simulink model "Main_Sim_test_rwafail_mtqfail"  (R2018b)
settings: Solver=FixedStepAuto  StartTime=0.0  StopTime=30000  FixedStep=simParams.sample_time_s  RelTol=1e-3  EnableMultiTasking=on
undefined symbols (not defined in the file): FSW_Lib
libraries: actuators_lib x1, CDH_command_lib x1, Environment_lib x1, MEKF_SensorCheck_Lib x1, actuator_processing_lib x1, allocation_lib x1, control_command_generation_lib x1, evironmentEstimation_lib x1, mode_select_lib x1, target_gen_lib x1, Sensors_Lib x1, satelliteDynamics_lib x1
settings Model: Creator=devantormey  LastModifiedBy=colem
settings OptimizationCC: LifeSpan=inf
settings DebuggingCC: SFUnexpectedBacktrackingDiag=warning  SFNoUnconditionalDefaultTransitionDiag=warning
settings SFSimCC: SimUseLocalCustomCode=off
settings RTWCC: RTWUseLocalCustomCode=off
settings CodeAppCC: StateflowObjectComments=on
settings GRTTargetCC: TargetLangStandard=C89/C90 (ANSI)  GeneratePreprocessorConditionals=Disable all
settings ConfigComp: CovMetricSettings=dw  CovHtmlReporting=on  CovSaveCumulativeToWorkspaceVar=on  CovSaveSingleToWorkspaceVar=on  CovExternalEMLEnable=off

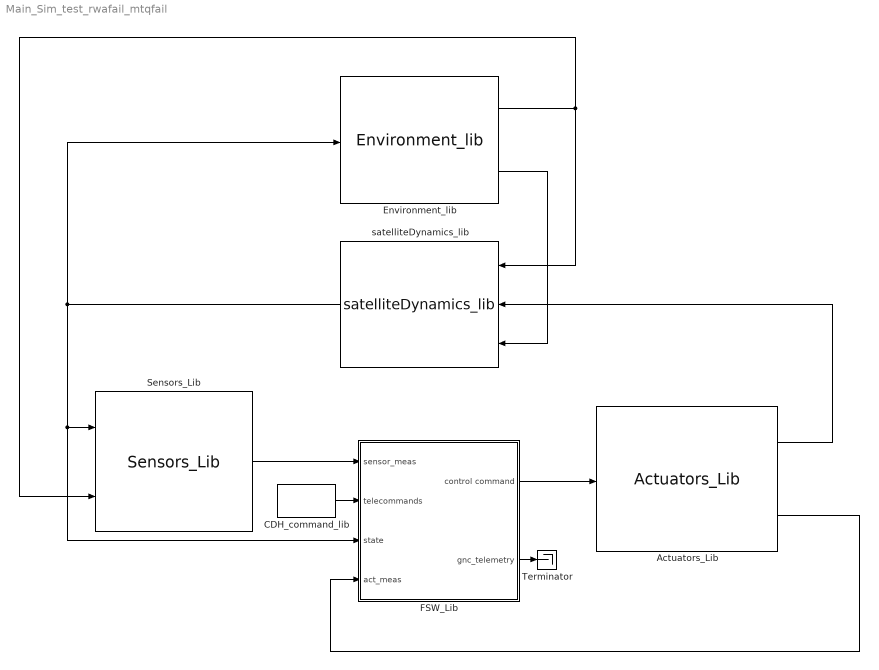
== system Main_Sim_test_rwafail_mtqfail ==
  Actuators_Lib : actuators_lib/Actuators_Lib  SystemSampleTime=-1
  CDH_command_lib : CDH_command_lib/CDH_command_lib  SystemSampleTime=-1
  Environment_lib : Environment_lib/Environment_lib  SystemSampleTime=-1
  FSW_Lib : Subsystem  AncestorBlock=FSW_Lib/FSW_Lib
  Sensors_Lib : Sensors_Lib/Sensors_Lib  SystemSampleTime=-1
      link override Goto3: GotoTag=B_eci_T
  Terminator : Terminator
  satelliteDynamics_lib : satelliteDynamics_lib/satelliteDynamics_lib  SystemSampleTime=-1
      link override "RigidBodyDynamics/Discrete-Time Integrator ": InitialCondition=simParams.initialConditions.w0
  wires:
  FSW_Lib/1(control command) -> Actuators_Lib/1
  Sensors_Lib/1 -> FSW_Lib/1(sensor_meas)
  satelliteDynamics_lib/1 -> Environment_lib/1, FSW_Lib/3(state), Sensors_Lib/1
  Environment_lib/1 -> Sensors_Lib/2, satelliteDynamics_lib/1
  Actuators_Lib/1 -> satelliteDynamics_lib/2
  FSW_Lib/2(gnc_telemetry) -> Terminator/1
  CDH_command_lib/1 -> FSW_Lib/2(telecommands)
  Environment_lib/2 -> satelliteDynamics_lib/3
  Actuators_Lib/2 -> FSW_Lib/4(act_meas)

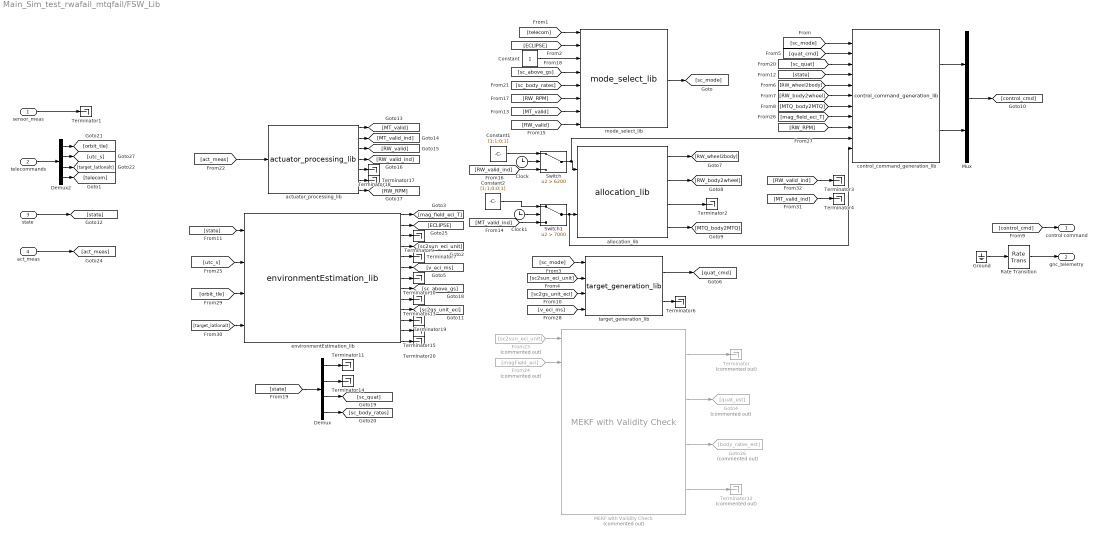
== system Main_Sim_test_rwafail_mtqfail/FSW_Lib ==
  sensor_meas : Inport
  telecommands : Inport  Port=2
  state : Inport  Port=3
  act_meas : Inport  Port=4
  Clock : Clock
  Clock1 : Clock
  Constant : Constant
  Constant1 : Constant  Value=[1;1;0;1]
  Constant2 : Constant  Value=[1;1;0;0;1]
  Demux : Demux  Outputs=[3 3 4 3]
  Demux2 : Demux  Outputs=[9 1 3 7]
  From23 : From  Commented=on  GotoTag=sc2sun_eci_unit
  From24 : From  Commented=on  GotoTag=magField_eci
  Goto26 : Goto  Commented=on  GotoTag=body_rates_est
  Goto4 : Goto  Commented=on  GotoTag=quat_est
  Ground : Ground
  MEKF with Validity Check : MEKF_SensorCheck_Lib/MEKF with Validity Check  Commented=on  SystemSampleTime=-1
  Mux : Mux  Inputs=[4 5]
  Rate Transition : RateTransition  OutPortSampleTime=fswParams.sample_time_s
  Switch : Switch  Criteria=u2 > Threshold  Threshold=6200
  Switch1 : Switch  Criteria=u2 > Threshold  Threshold=7000
  Terminator : Terminator  Commented=on
  Terminator{1..4,6..7,9..11,13..15,17..20} (16 alike) : Terminator
  Terminator12 : Terminator  Commented=on
  actuator_processing_lib : actuator_processing_lib/actuator_processing_lib  SystemSampleTime=-1
  allocation_lib : allocation_lib/allocation_lib  SystemSampleTime=-1
  control_command_generation_lib : control_command_generation_lib/control_command_generation_lib  SystemSampleTime=-1
  environmentEstimation_lib : evironmentEstimation_lib/environmentEstimation_lib  SystemSampleTime=-1
  mode_select_lib : mode_select_lib/mode_select_lib  SystemSampleTime=-1
  target_generation_lib : target_gen_lib/target_generation_lib  SystemSampleTime=-1
  control command : Outport
  gnc_telemetry : Outport  Port=2
  wires:
  [MT_valid_ind] -> Terminator4/1
  [RW_valid_ind] -> Terminator3/1
  Rate Transition/1 -> gnc_telemetry/1
  target_generation_lib/1 -> [quat_cmd]
  [target_latlonalt] -> environmentEstimation_lib/4
  Demux2/3 -> [target_latlonalt]
  Demux2/1 -> [orbit_tle]
  [v_eci_ms] -> target_generation_lib/4
  [RW_RPM] -> control_command_generation_lib/9
  [mag_field_eci_T] -> control_command_generation_lib/8
  Demux2/2 -> [utc_s]
  Demux2/4 -> [telecom]
  MEKF with Validity Check/2 -> Goto4/1
  MEKF with Validity Check/3 -> Goto26/1
  MEKF with Validity Check/4 -> Terminator12/1
  MEKF with Validity Check/1 -> Terminator/1
  From24/1 -> MEKF with Validity Check/2
  From23/1 -> MEKF with Validity Check/1
  environmentEstimation_lib/11 -> Terminator19/1
  environmentEstimation_lib/13 -> Terminator20/1
  environmentEstimation_lib/12 -> Terminator15/1
  Demux/2 -> Terminator14/1
  Demux/1 -> Terminator11/1
  Demux/4 -> [sc_body_rates]
  Demux/3 -> [sc_quat]
  [state] -> Demux/1
  [act_meas] -> actuator_processing_lib/1
  actuator_processing_lib/7 -> [RW_RPM]
  actuator_processing_lib/6 -> Terminator17/1
  actuator_processing_lib/5 -> Terminator18/1
  actuator_processing_lib/4 -> [RW_valid_ind]
  actuator_processing_lib/3 -> [RW_valid]
  actuator_processing_lib/2 -> [MT_valid_ind]
  actuator_processing_lib/1 -> [MT_valid]
  act_meas/1 -> [act_meas]
  [state] -> control_command_generation_lib/4
  [state] -> environmentEstimation_lib/1
  state/1 -> [state]
  [sc2gs_unit_eci] -> target_generation_lib/3
  [orbit_tle] -> environmentEstimation_lib/3
  [utc_s] -> environmentEstimation_lib/2
  environmentEstimation_lib/10 -> [sc2gs_unit_eci]
  environmentEstimation_lib/9 -> Terminator13/1
  environmentEstimation_lib/8 -> [sc_above_gs]
  environmentEstimation_lib/7 -> Terminator10/1
  environmentEstimation_lib/6 -> [v_eci_ms]
  environmentEstimation_lib/5 -> Terminator7/1
  environmentEstimation_lib/4 -> [sc2sun_eci_unit]
  environmentEstimation_lib/3 -> Terminator9/1
  environmentEstimation_lib/2 -> [ECLIPSE]
  environmentEstimation_lib/1 -> [mag_field_eci_T]
  Mux/1 -> [control_cmd]
  control_command_generation_lib/1 -> Mux/1
  control_command_generation_lib/2 -> Mux/2
  [MTQ_body2MTQ] -> control_command_generation_lib/7
  [RW_body2wheel] -> control_command_generation_lib/6
  allocation_lib/4 -> [MTQ_body2MTQ]
  allocation_lib/3 -> Terminator2/1
  [RW_wheel2body] -> control_command_generation_lib/5
  allocation_lib/2 -> [RW_body2wheel]
  allocation_lib/1 -> [RW_wheel2body]
  [sc_quat] -> control_command_generation_lib/3
  [RW_valid_ind] -> Switch/3
  [quat_cmd] -> control_command_generation_lib/2
  target_generation_lib/2 -> Terminator6/1
  [sc2sun_eci_unit] -> target_generation_lib/2
  [sc_mode] -> target_generation_lib/1
  [RW_valid] -> mode_select_lib/8
  [MT_valid] -> mode_select_lib/7
  Constant/1 -> mode_select_lib/3
  [RW_RPM] -> mode_select_lib/6
  [sc_body_rates] -> mode_select_lib/5
  [sc_above_gs] -> mode_select_lib/4
  [ECLIPSE] -> mode_select_lib/2
  [telecom] -> mode_select_lib/1
  [sc_mode] -> control_command_generation_lib/1
  mode_select_lib/1 -> [sc_mode]
  [control_cmd] -> control command/1
  Ground/1 -> Rate Transition/1
  telecommands/1 -> Demux2/1
  sensor_meas/1 -> Terminator1/1
  Clock/1 -> Switch/2
  Constant1/1 -> Switch/1
  Switch/1 -> control_command_generation_lib/10, allocation_lib/1
  Constant2/1 -> Switch1/1
  [MT_valid_ind] -> Switch1/3
  Clock1/1 -> Switch1/2
  Switch1/1 -> control_command_generation_lib/11, allocation_lib/2
